simulink model "beam_PID"  (Simulink 7.7)
settings: Solver=ode15s  StartTime=0.0  StopTime=0.05  RelTol=1e-3
values from neighbouring files (symbols this model uses):
  d = 0.0300    (= 0.03)    [BEAm ball carac.m]    (also in Ball_Beam_Lead_PD.m = 0.05; bb_carac.m)
  g = 9.8000    (= 9.8)    [BEAm ball carac.m]    (also in Ball_Beam_Lead_PD.m = -9.8; bb_carac.m = -9.8)
  J = 2/5*m*R^2    (= 3.42e-06)    [BEAm ball carac.m]    (also in Ball_Beam_Lead_PD.m = 1e-06; bb_carac.m)
  L = 0.4300    (= 0.43)    [BEAm ball carac.m]    (also in Ball_Beam_Lead_PD.m = 1; bb_carac.m)
  m = 38*10^-3    (= 0.038)    [BEAm ball carac.m]    (also in Ball_Beam_Lead_PD.m = 0.15; bb_carac.m)
  R = 0.0150    (= 0.015)    [BEAm ball carac.m]    (also in Ball_Beam_Lead_PD.m; bb_carac.m)
libraries: simulink x1
settings Model: Creator=XnL  LastModifiedBy=XnL
settings DataIOCC: SaveState=on

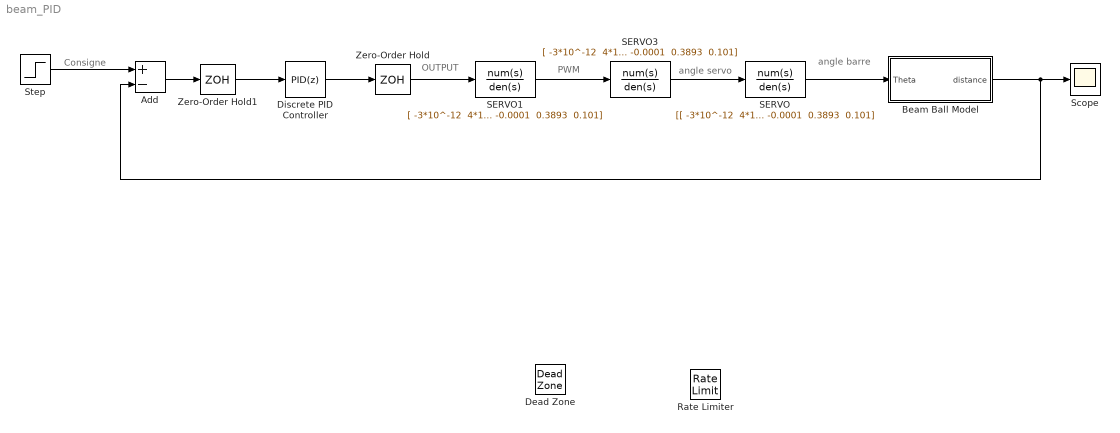
== system beam_PID ==
  note: angle barre
  note: angle servo
  note: PWM
  note: OUTPUT
  note: Consigne
  Add : Sum  Inputs=+-
  Beam Ball Model : Subsystem
  Dead Zone : DeadZone  SaturateOnIntegerOverflow=on
  Discrete PID Controller : simulink/Continuous/PID Controller  SystemSampleTime=-1  Controller=PID  TimeDomain=Discrete-time  SampleTime=10^-3  IntegratorMethod=Forward Euler  FilterMethod=Forward Euler  Form=Parallel  P=1  I=1  D=1  N=2  InitialConditionSource=internal  InitialConditionForIntegrator=0  InitialConditionForFilter=0  ExternalReset=none  LimitOutput=off  UpperSaturationLimit=inf  LowerSaturationLimit=-inf  LinearizeAsGain=off  AntiWindupMode=none  Kb=1  TrackingMode=off  Kt=1  PParamMin=[]  PParamMax=[]  IParamMin=[]  IParamMax=[]  DParamMin=[]  DParamMax=[]  NParamMin=[]  NParamMax=[]  KbParamMin=[]  KbParamMax=[]  KtParamMin=[]  KtParamMax=[]  POutMin=[]  POutMax=[]  IOutMin=[]  IOutMax=[]  DOutMin=[]  DOutMax=[]  NOutMin=[]  NOutMax=[]  KbOutMin=[]  KbOutMax=[]  KtOutMin=[]  KtOutMax=[]  IntegratorOutMin=[]  IntegratorOutMax=[]  FilterOutMin=[]  FilterOutMax=[]  SumOutMin=[]  SumOutMax=[]  SumI1OutMin=[]  SumI1OutMax=[]  SumI2OutMin=[]  SumI2OutMax=[]  SumI3OutMin=[]  SumI3OutMax=[]  SumDOutMin=[]  SumDOutMax=[]  SaturationOutMin=[]  SaturationOutMax=[]  IntegratorContinuousStateAttributes=''  IntegratorStateMustResolveToSignalObject=off  IntegratorRTWStateStorageClass=Auto  FilterContinuousStateAttributes=''  FilterStateMustResolveToSignalObject=off  FilterRTWStateStorageClass=Auto
  Rate Limiter : RateLimiter  SampleTimeMode=inherited
  SERVO : TransferFcn  Numerator="[[ -3*10^-12  4*10^-10  10^-07  2*10^-5   -0.0001  0.3893  0.101]]"  Denominator="[ -3*10^-12  4*10^-10  10^-07  2*10^-5   -0.0001  0.3893  0.101]"
  SERVO1 : TransferFcn  Numerator="[ -3*10^-12  4*10^-10  10^-07  2*10^-5   -0.0001  0.3893  0.101]"  Denominator="[ -3*10^-12  4*10^-10  10^-07  2*10^-5   -0.0001  0.3893  0.101]"
  SERVO3 : TransferFcn  Numerator="[ -3*10^-12  4*10^-10  10^-07  2*10^-5   -0.0001  0.3893  0.101]"  Denominator="[ -3*10^-12  4*10^-10  10^-07  2*10^-5   -0.0001  0.3893  0.101]"
  Scope : Scope
  Step : Step  Time=0  After=220  SampleTime=0
  Zero-Order Hold : ZeroOrderHold
  Zero-Order Hold1 : ZeroOrderHold
  wires:
  SERVO/1 -> Beam Ball Model/1(Theta)
  SERVO3/1 -> SERVO/1
  SERVO1/1 -> SERVO3/1
  Zero-Order Hold/1 -> SERVO1/1
  Discrete PID Controller/1 -> Zero-Order Hold/1
  Zero-Order Hold1/1 -> Discrete PID Controller/1
  Beam Ball Model/1(distance) -> Scope/1, Add/2
  Add/1 -> Zero-Order Hold1/1
  Step/1 -> Add/1

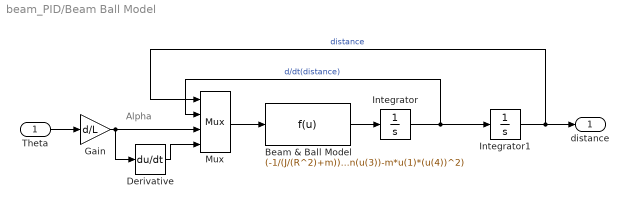
== system beam_PID/Beam Ball Model ==
  note: Alpha
  Theta : Inport
  Beam & Ball Model : Fcn  Expr=(-1/(J/(R^2)+m))*(m*g*sin(u(3))-m*u(1)*(u(4))^2)
  Derivative : Derivative
  Gain : Gain  Gain=d/L
  Integrator : Integrator
  Integrator1 : Integrator
  Mux : Mux
  distance : Outport
  wires:
  Integrator/1 -> Integrator1/1, Mux/2  "d/dt(distance)"
  Integrator1/1 -> distance/1, Mux/1  "distance"
  Beam & Ball Model/1 -> Integrator/1
  Mux/1 -> Beam & Ball Model/1
  Gain/1 -> Derivative/1, Mux/3
  Derivative/1 -> Mux/4
  Theta/1 -> Gain/1
